simulink model "Tractor_Trailer_Flatness_Simulation"  (R2022b)
settings: Solver=ode4  StartTime=0.01  StopTime=20  FixedStep=0.01  RelTol=1e-3
InitFcn:
  | d0 = 1;
  | Dt=0.01;
  | 
  | %% if we want to "externalise" the trailer link from the car
  | a = 1.5;
  | 
  | %% distance between car and trailer
  | b = 2.5;
  | 
  | d1=b;
  | 
  | delay = 0.01;
  | 
  | %% delay with 0 signal before (to avoid instabilities before the "real" path following simulation")
  | del=2;
  | 
  | %% delay to sub above to chose starting using real value
  | dedel=1;
  | 
  | y0 = 0;
  | x0 = d1;
  | co=0;
  | 
  | the_pre=0;
  | the_pre_pre=0;
  | sdt=0.01;
  | 
  | ti_mod = 0.3;
  | 
  | phi0=pi;
  | 
  | %% Backward= pi, forward = 0
  | for_back=pi;
  | %%
  | 
  | %% Circle initial conditons forward
  | % for_back=0;
  | % dedel = 1.5;
  | % x_dot_init = 0;
  | % y_dot_init = 3;
  | % x_init = 0;
  | % y_init = 0;
  | % x0_init = b + del-dedel;
  | % y0_init = 0;
  | % theta0_init=for_back;
  | % theta1_init=0;
  | 
  | %% Circle initial conditons backward
  | % for_back=pi;
  | % dedel = 1.5;
  | % x_dot_init = 0;
  | % y_dot_init = 3;
  | % x_init = 0;
  | % y_init = 0;
  | % x0_init = -b;
  | % y0_init = 0;
  | % theta0_init=for_back;
  | % theta1_init=0;
  | 
  | %% func1 initial conditons
  | % x_dot_init = 1;
  | % y_dot_init = 0;
  | % x_init = 0;
  | % y_init = 0;
  | % x0_init = 0;
  | % y0_init = 0;
  | % theta0_init=0;
  | % theta1_init=0;
  | 
  | %% Wavy_up initial conditons
  | % x_dot_init = 0;
  | % y_dot_init = 0;
  | % x_init = 0;
  | % y_init = 0;
  | % x0_init = 0;
  | % y0_init = 0;
  | % theta0_init=0;
  | % theta1_init=0;
  | 
  | %% Backward Initial conditons for waving upward
  | % for_back=pi;
  | % x_dot_init = 1;
  | % y_dot_init = 0;
  | %
  | % x_init = 0;
  | % y_init = 0;
  | %
  | % %plant init
  | % x0_init = -b;
  | % y0_init = 0;
  | % theta0_init=for_back;
  | % theta1_init=0;
  | % del=pi;
  | 
  | %% Forward Initial conditons for waving upward
  | for_back=0;
  | x_dot_init = 1;
  | y_dot_init = 0;
  | 
  | x_init = 0;
  | y_init = 0;
  | 
  | %plant init
  | x0_init = b;
  | y0_init = 0;
  | theta0_init=for_back;
  | theta1_init=0;
  | del=pi;
  | 
  | 
  | %% Forward initial conditons for exp
  | % dedel=del;
  | % for_back=0;
  | % x_dot_init = 1;
  | % y_dot_init = 0;
  | % x_init = 0;
  | % y_init = 0;
  | % x0_init = 0;
  | % y0_init = 0;
  | % theta0_init=for_back;
  | % theta1_init=0;
  | 
  | %% Backward initial conditons for exp
  | % dedel=del-0.2;
  | % for_back=pi;
  | % x_dot_init = 1;
  | % y_dot_init = 0;
  | % x_init = 0;
  | % y_init = 0;
  | % x0_init = -b;
  | % y0_init = 0;
  | % theta0_init=for_back;
  | % theta1_init=0;
  | 
  | 
  | %% Cosinus initial conditons forward
  | % for_back=0;
  | % dedel=1;
  | % x_dot_init = 3;
  | % y_dot_init = 0;
  | % x_init = 0;
  | % y_init = 0;
  | % x0_init = b;
  | % y0_init = 0;
  | % theta0_init=for_back;
  | % theta1_init=0;
  | 
  | %% Cosinus initial conditons backward
  | % for_back=pi;
  | % dedel=1;
  | % x_dot_init = 3;
  | % y_dot_init = 0;
  | % x_init = 0;
  | % y_init = 0;
  | % x0_init = -b;
  | % y0_init = 0;
  | % theta0_init=for_back;
  | % theta1_init=0;
settings Model: Creator=chaudhuri  LastModifiedBy=Tugdual
settings ModelReferenceCC: EnableRefExpFcnMdlSchedulingChecks=on

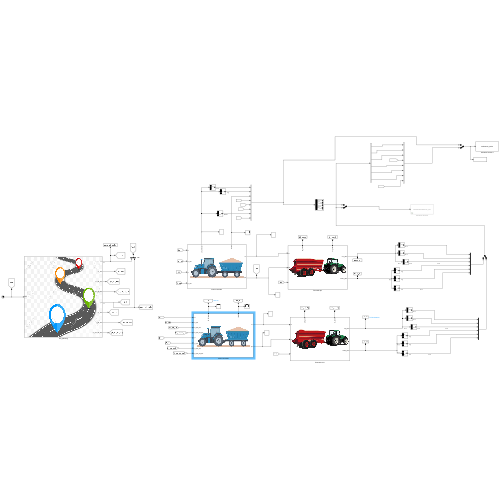
[thumbnail: Simulink's stored preview of the top-level diagram]
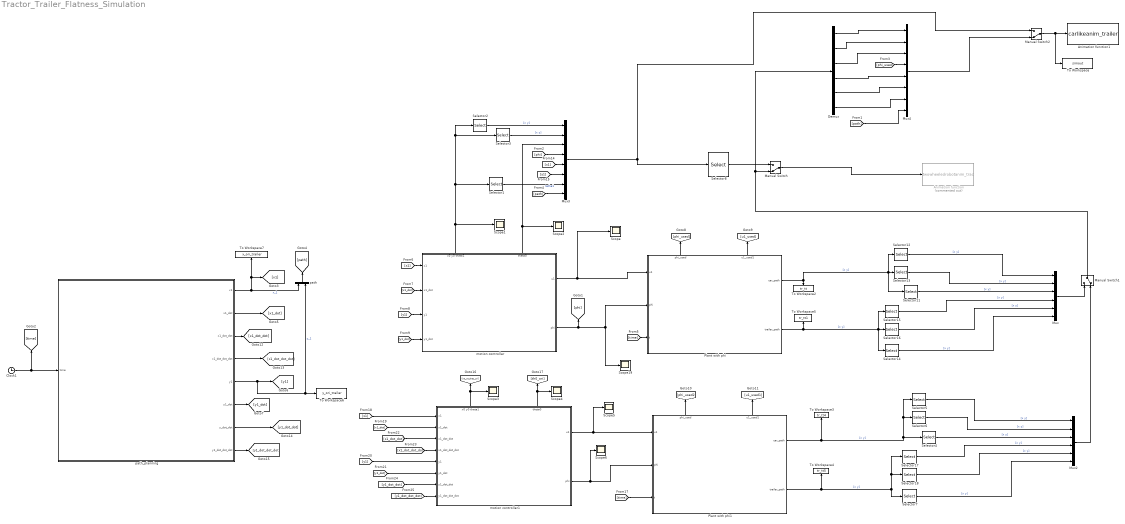
== system Tractor_Trailer_Flatness_Simulation ==
  Animation function : S-Function  Commented=on  FunctionName=twowheeledrobotanim_trac  SFunctionDeploymentMode=off  EnableBusSupport=off
  Animation function1 : S-Function  FunctionName=carlikeanim_trailer  SFunctionDeploymentMode=off  EnableBusSupport=off
  Clock1 : Clock
  Demux : Demux  Outputs=6
  Manual Switch : ManualSwitch  CurrentSetting=0
  Manual Switch1 : ManualSwitch  CurrentSetting=0
  Manual Switch2 : ManualSwitch  CurrentSetting=0
  Mux : Mux  Inputs=6
  Mux2 : Mux  Inputs=6
  Mux3 : Mux  Inputs=8
  Mux4 : Mux  Inputs=8
  Plant with phi : Subsystem
      settings: PortSchema="{\"entries\":[{\"content\":{\"sides\":[{\"content\":{\"connectorIds\":[\"In1\",\"In2\",\"In3\"]},\"type\":\"ConnectorPlacement.EquallySpacedRectSide\",\"uuid\":\"e7db4861-1c7b-44d0-8ae0-043891a2d65e\"},{\"content\":{\"connectorIds\":[\"Out1\",\"Out2\"],\"side\":\"RIGHT\"},\"type\":\"ConnectorPlacement.EquallySpacedRectSide\",\"uuid\":\"ca6953ca-f3e9-441a-9b66-bf77f2babfba\"},{\"content\":{\"connectorIds\":[\"Out3\",\"Out4\"],\"side\":\"TOP\"},\"type\":\"ConnectorPlacement.EquallySpacedRectSide\",\"uuid\":\"0653e744-f46f-49ca-b3b7-6a2721aef055\"}]},\"type\":\"ConnectorPlacement.EquallySpacedConnector\",\"uuid\":\"d05efadf-1bd4-4ab0-9eff-99e9b7844dfa\"}],\"packageUris\":[\"http://schema.mathworks.com/mf0/Connector/R2020b\"],\"version\":\"1.0\"}"
      mask Display: image('$imagefile'); % Use "Edit Image" on toolstrip to change.
  Plant with phi1 : Subsystem
      settings: PortSchema="{\"entries\":[{\"content\":{\"sides\":[{\"content\":{\"connectorIds\":[\"In1\",\"In2\",\"In3\"]},\"type\":\"ConnectorPlacement.EquallySpacedRectSide\",\"uuid\":\"e7db4861-1c7b-44d0-8ae0-043891a2d65e\"},{\"content\":{\"connectorIds\":[\"Out1\",\"Out2\"],\"side\":\"RIGHT\"},\"type\":\"ConnectorPlacement.EquallySpacedRectSide\",\"uuid\":\"ca6953ca-f3e9-441a-9b66-bf77f2babfba\"},{\"content\":{\"connectorIds\":[\"Out3\",\"Out4\"],\"side\":\"TOP\"},\"type\":\"ConnectorPlacement.EquallySpacedRectSide\",\"uuid\":\"0653e744-f46f-49ca-b3b7-6a2721aef055\"}]},\"type\":\"ConnectorPlacement.EquallySpacedConnector\",\"uuid\":\"d05efadf-1bd4-4ab0-9eff-99e9b7844dfa\"}],\"packageUris\":[\"http://schema.mathworks.com/mf0/Connector/R2020b\"],\"version\":\"1.0\"}"
      mask Display: image('$imagefile'); % Use "Edit Image" on toolstrip to change.
  Scope{,1..6,19} (8 alike) : Scope
  Selector{1,4,7,11,14} (5 alike) : Selector  InputPortWidth=3  IndexOptions=Index vector (dialog)  Indices=[3]  OutputSizes=1
  Selector{2,5,12,15,17} (5 alike) : Selector  InputPortWidth=3  IndexOptions=Index vector (dialog)  Indices=[1]  OutputSizes=1
  Selector{3,6,13,16,18} (5 alike) : Selector  InputPortWidth=3  IndexOptions=Index vector (dialog)  Indices=[2]  OutputSizes=1
  Selector8 : Selector  InputPortWidth=9  IndexOptions=Index vector (dialog)  Indices=[1 2 3 5 6 7]  OutputSizes=1
  To Workspace : ToWorkspace  VariableName=simout  SaveFormat=Timeseries  SampleTime=-1
  To Workspace2 : ToWorkspace  VariableName=tr_tt  SaveFormat=Timeseries  SampleTime=-1
  To Workspace3 : ToWorkspace  VariableName=tr_tt4  SaveFormat=Timeseries  SampleTime=-1
  To Workspace4 : ToWorkspace  VariableName=tr_tt5  SaveFormat=Timeseries  SampleTime=-1
  To Workspace5 : ToWorkspace  VariableName=tr_tt1  SaveFormat=Timeseries  SampleTime=-1
  To Workspace6 : ToWorkspace  VariableName=y_ori_trailer  SaveFormat=Timeseries  SampleTime=-1
      settings: Save2DSignal=2-D array (concatenate along first dimension)
  To Workspace7 : ToWorkspace  VariableName=x_ori_trailer  SaveFormat=Timeseries  SampleTime=-1
      settings: Save2DSignal=2-D array (concatenate along first dimension)
  motion controller : Subsystem
      settings: PortSchema="{\"entries\":[{\"content\":{\"sides\":[{\"content\":{\"connectorIds\":[\"In1\",\"In2\",\"In3\",\"In4\"]},\"type\":\"ConnectorPlacement.EquallySpacedRectSide\",\"uuid\":\"11bc3301-7ab6-4d38-8445-7de1e6050525\"},{\"content\":{\"connectorIds\":[\"Out1\",\"Out2\"],\"side\":\"RIGHT\"},\"type\":\"ConnectorPlacement.EquallySpacedRectSide\",\"uuid\":\"374bee85-8743-45f2-a60a-268bfdaad2ec\"},{\"content\":{\"connectorIds\":[\"Out3\",\"Out4\"],\"side\":\"TOP\"},\"type\":\"ConnectorPlacement.EquallySpacedRectSide\",\"uuid\":\"71c6a0a5-27e8-424b-8871-57b58ecd48a6\"}]},\"type\":\"ConnectorPlacement.EquallySpacedConnector\",\"uuid\":\"fb4e8639-9b4e-4508-bb82-15087a60f723\"}],\"packageUris\":[\"http://schema.mathworks.com/mf0/Connector/R2020b\"],\"version\":\"1.0\"}"
      mask Display: image('$imagefile'); % Use "Edit Image" on toolstrip to change.
  motion controller1 : Subsystem
      settings: PortSchema="{\"entries\":[{\"content\":{\"sides\":[{\"content\":{\"connectorIds\":[\"In1\",\"In2\",\"In3\",\"In4\",\"In5\",\"In6\",\"In7\",\"In8\"]},\"type\":\"ConnectorPlacement.EquallySpacedRectSide\",\"uuid\":\"11bc3301-7ab6-4d38-8445-7de1e6050525\"},{\"content\":{\"connectorIds\":[\"Out1\",\"Out2\"],\"side\":\"RIGHT\"},\"type\":\"ConnectorPlacement.EquallySpacedRectSide\",\"uuid\":\"374bee85-8743-45f2-a60a-268bfdaad2ec\"},{\"content\":{\"connectorIds\":[\"Out3\",\"Out4\"],\"side\":\"TOP\"},\"type\":\"ConnectorPlacement.EquallySpacedRectSide\",\"uuid\":\"71c6a0a5-27e8-424b-8871-57b58ecd48a6\"}]},\"type\":\"ConnectorPlacement.EquallySpacedConnector\",\"uuid\":\"fb4e8639-9b4e-4508-bb82-15087a60f723\"}],\"packageUris\":[\"http://schema.mathworks.com/mf0/Connector/R2020b\"],\"version\":\"1.0\"}"
      mask Display: image('$imagefile'); % Use "Edit Image" on toolstrip to change.
  path : Mux  Inputs=2
  path_planning : Subsystem
      mask Display: image('$imagefile'); % Use "Edit Image" on toolstrip to change.
  wires:
  Clock1/1 -> [time], path_planning/1(time)
  motion controller/2(phi) -> [phi], Plant with phi/2(phi), Scope19/1
  Plant with phi/1(car_path) -> Selector11/1, Selector12/1, Selector13/1, To Workspace2/1  "[x y]"
  Selector11/1 -> Mux/3  "[x y]"
  Selector12/1 -> Mux/1  "[x y]"
  Selector13/1 -> Mux/2  "[x y]"
  Selector16/1 -> Mux/5  "[x y]"
  Selector15/1 -> Mux/4  "[x y]"
  Plant with phi/2(trailer_path) -> Selector14/1, Selector15/1, Selector16/1, To Workspace5/1  "[x y]"
  Selector14/1 -> Mux/6  "[x y]"
  Manual Switch1/1 -> Demux/1, Manual Switch/2
  motion controller/1(u1) -> Plant with phi/1(u1), Scope/1
  motion controller/3(x0 y0 theta1) -> Scope1/1, Selector2/1, Selector3/1, Selector1/1
  Selector1/1 -> Mux3/7  "tetha1"
  Selector3/1 -> Mux3/2  "[x y]"
  Selector2/1 -> Mux3/1  "[x y]"
  Selector17/1 -> Mux2/4  "[x y]"
  Selector7/1 -> Mux2/6  "[x y]"
  Plant with phi1/2(trailer_path) -> To Workspace4/1, Selector18/1, Selector17/1, Selector7/1  "[x y]"
  Selector18/1 -> Mux2/5  "[x y]"
  Plant with phi1/1(car_path) -> Selector4/1, Selector5/1, Selector6/1, To Workspace3/1  "[x y]"
  Selector6/1 -> Mux2/2  "[x y]"
  Selector5/1 -> Mux2/1  "[x y]"
  Mux2/1 -> Manual Switch1/2
  Selector4/1 -> Mux2/3  "[x y]"
  Mux/1 -> Manual Switch1/1
  Manual Switch2/1 -> To Workspace/1, Animation function1/1
  Manual Switch/1 -> Animation function/1
  motion controller/4(theta0) -> Scope2/1, Mux3/3
  Mux4/1 -> Manual Switch2/2
  Mux3/1 -> Selector8/1, Manual Switch2/1
  Demux/1 -> Mux4/1
  Demux/2 -> Mux4/2
  Demux/3 -> Mux4/3
  Demux/4 -> Mux4/5
  Demux/5 -> Mux4/6
  Demux/6 -> Mux4/7
  path/1 -> [path]
  [path] -> Mux4/8
  [phi] -> Mux3/4
  [phi_used] -> Mux4/4
  [path] -> Mux3/8
  [time] -> Plant with phi/3(t)
  Selector8/1 -> Manual Switch/1
  [x1] -> Mux3/5
  [y1] -> Mux3/6
  [x1] -> motion controller/1(x1)
  [x1_dot] -> motion controller/2(x1_dot)
  [y1] -> motion controller/3(y1)
  [y1_dot] -> motion controller/4(y1_dot)
  path_planning/6(y1_dot) -> [y1_dot]
  path_planning/5(y1) -> To Workspace6/1, path/2, [y1]  "y_1"
  path_planning/2(x1_dot) -> [x1_dot]
  path_planning/1(x1) -> path/1, [x1], To Workspace7/1  "x_1"
  Plant with phi/3(phi_used) -> [phi_used]
  Plant with phi/4(u1_used1) -> [u1_used]
  motion controller1/1(u1) -> Scope5/1, Plant with phi1/1(u1)
  motion controller1/2(phi) -> Scope6/1, Plant with phi1/2(phi)
  [time] -> Plant with phi1/3(t)
  [x1_dot_dot] -> motion controller1/3(x1_dot_dot)
  [x1_dot] -> motion controller1/2(x1_dot)
  [x1] -> motion controller1/1(x1)
  [y1] -> motion controller1/5(y1)
  [y1_dot] -> motion controller1/6(y1_dot)
  [y1_dot_dot] -> motion controller1/7(y1_dot_dot)
  [y1_dot_dot_dot] -> motion controller1/8(y1_dot_dot_dot)
  [x1_dot_dot_dot] -> motion controller1/4(x1_dot_dot_dot)
  motion controller1/4(theta0) -> [th0_ori], Scope4/1
  motion controller1/3(x0 y0 theta1) -> Scope3/1, [x0_y0_the1_ori]
  Plant with phi1/4(u1_used1) -> [u1_used1]
  Plant with phi1/3(phi_used) -> [phi_used2]
  path_planning/8(y1_dot_dot_dot) -> [y1_dot_dot_dot]
  path_planning/7(y_dot_dot) -> [y1_dot_dot]
  path_planning/4(x1_dot_dot_dot) -> [x1_dot_dot_dot]
  path_planning/3(x1_dot_dot) -> [x1_dot_dot]

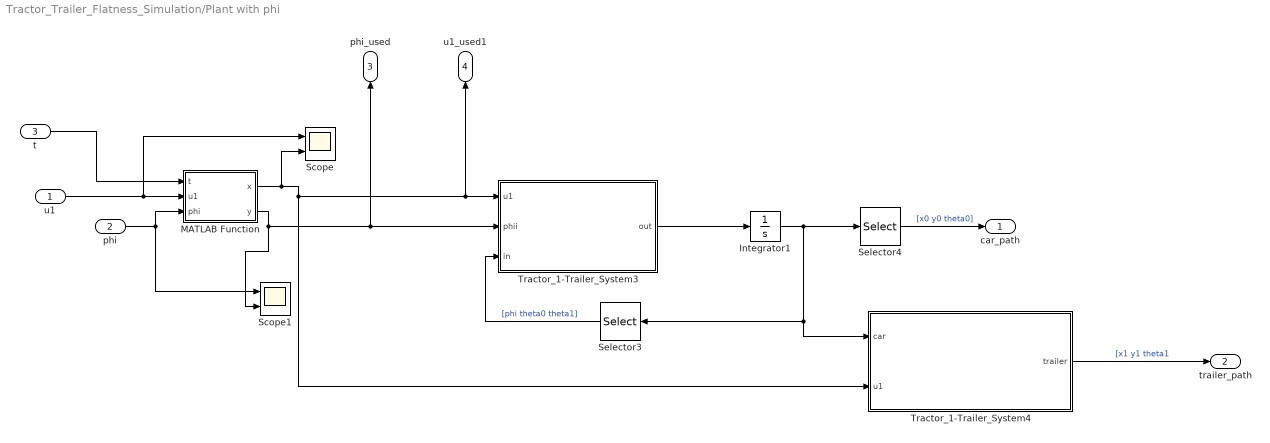
== system Tractor_Trailer_Flatness_Simulation/Plant with phi ==
  u1 : Inport
  phi : Inport  Port=2
  t : Inport  Port=3
  Integrator1 : Integrator  InitialCondition=[x0_init;y0_init;theta0_init;theta1_init]
  MATLAB Function : MATLAB Function  TreatAsAtomicUnit=on
  Scope : Scope  NumInputPorts=2
  Scope1 : Scope  NumInputPorts=2
  Selector3 : Selector  InputPortWidth=4  IndexOptions=Index vector (dialog)  Indices=[3 4]  OutputSizes=1
  Selector4 : Selector  InputPortWidth=4  IndexOptions=Index vector (dialog)  Indices=[1 2 3]  OutputSizes=1
  Tractor_1-Trailer_System3 : MATLAB Function  TreatAsAtomicUnit=on
  Tractor_1-Trailer_System4 : MATLAB Function  TreatAsAtomicUnit=on
  car_path : Outport
  trailer_path : Outport  Port=2
  phi_used : Outport  Port=3
  u1_used1 : Outport  Port=4
  wires:
  Tractor_1-Trailer_System4/1(trailer) -> trailer_path/1  "[x1 y1 theta1"
  Tractor_1-Trailer_System3/1(out) -> Integrator1/1
  Integrator1/1 -> Selector4/1, Tractor_1-Trailer_System4/1(car), Selector3/1
  Selector3/1 -> Tractor_1-Trailer_System3/3(in)  "[phi theta0 theta1]"
  Selector4/1 -> car_path/1  "[x0 y0 theta0]"
  MATLAB Function/2(y) -> Scope1/2, Tractor_1-Trailer_System3/2(phii), phi_used/1
  MATLAB Function/1(x) -> Scope/2, u1_used1/1, Tractor_1-Trailer_System3/1(u1), Tractor_1-Trailer_System4/2(u1)
  t/1 -> MATLAB Function/1(t)
  u1/1 -> Scope/1, MATLAB Function/2(u1)
  phi/1 -> Scope1/1, MATLAB Function/3(phi)

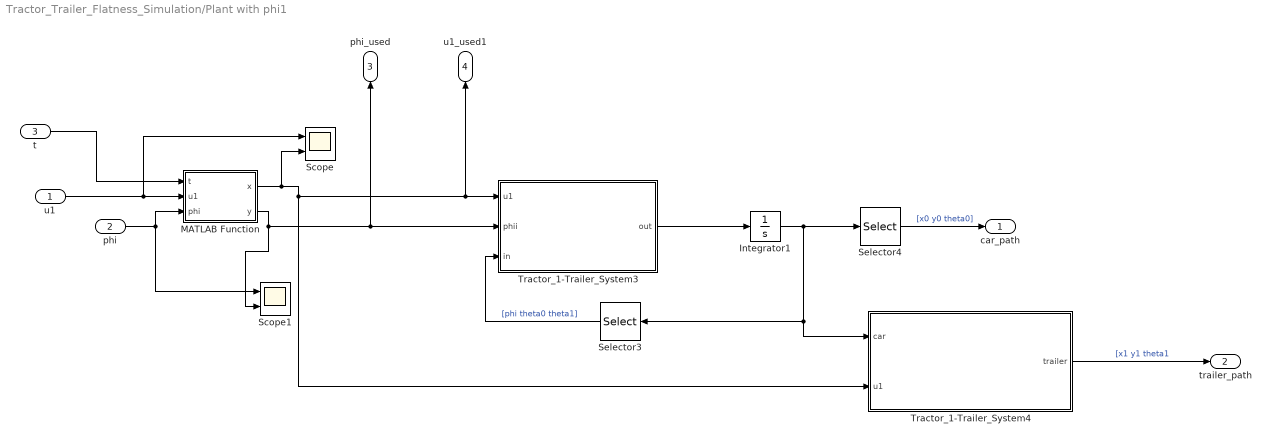
== system Tractor_Trailer_Flatness_Simulation/Plant with phi1 ==
  u1 : Inport
  phi : Inport  Port=2
  t : Inport  Port=3
  Integrator1 : Integrator  InitialCondition=[x0_init;y0_init;theta0_init;theta1_init]
  MATLAB Function : MATLAB Function  TreatAsAtomicUnit=on
  Scope : Scope  NumInputPorts=2
  Scope1 : Scope  NumInputPorts=2
  Selector3 : Selector  InputPortWidth=4  IndexOptions=Index vector (dialog)  Indices=[3 4]  OutputSizes=1
  Selector4 : Selector  InputPortWidth=4  IndexOptions=Index vector (dialog)  Indices=[1 2 3]  OutputSizes=1
  Tractor_1-Trailer_System3 : MATLAB Function  TreatAsAtomicUnit=on
  Tractor_1-Trailer_System4 : MATLAB Function  TreatAsAtomicUnit=on
  car_path : Outport
  trailer_path : Outport  Port=2
  phi_used : Outport  Port=3
  u1_used1 : Outport  Port=4
  wires:
  Tractor_1-Trailer_System4/1(trailer) -> trailer_path/1  "[x1 y1 theta1"
  Tractor_1-Trailer_System3/1(out) -> Integrator1/1
  Integrator1/1 -> Selector4/1, Tractor_1-Trailer_System4/1(car), Selector3/1
  Selector3/1 -> Tractor_1-Trailer_System3/3(in)  "[phi theta0 theta1]"
  Selector4/1 -> car_path/1  "[x0 y0 theta0]"
  MATLAB Function/2(y) -> Scope1/2, Tractor_1-Trailer_System3/2(phii), phi_used/1
  MATLAB Function/1(x) -> Scope/2, u1_used1/1, Tractor_1-Trailer_System3/1(u1), Tractor_1-Trailer_System4/2(u1)
  t/1 -> MATLAB Function/1(t)
  u1/1 -> Scope/1, MATLAB Function/2(u1)
  phi/1 -> Scope1/1, MATLAB Function/3(phi)

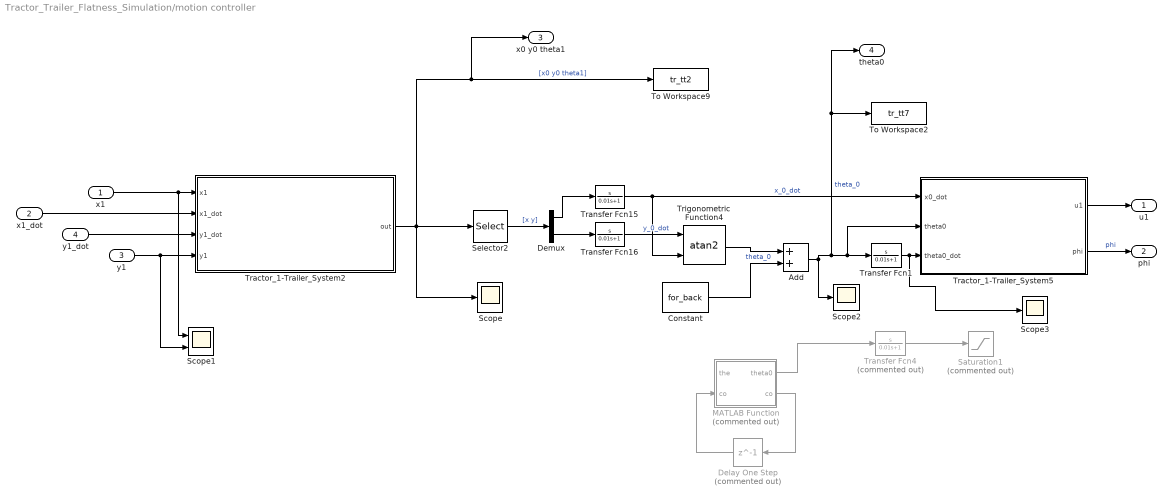
== system Tractor_Trailer_Flatness_Simulation/motion controller ==
  x1 : Inport
  x1_dot : Inport  Port=2
  y1 : Inport  Port=3
  y1_dot : Inport  Port=4
  Add : Sum
  Constant : Constant  Value=for_back
  Delay One Step : Delay  Commented=on  DelayLength=1
  Demux : Demux  Outputs=2
  MATLAB Function : MATLAB Function  Commented=on  TreatAsAtomicUnit=on
  Saturation1 : Saturate  Commented=on  UpperLimit=pi/4  LowerLimit=-pi/4
  Scope : Scope
  Scope1 : Scope  NumInputPorts=2
  Scope2 : Scope
  Scope3 : Scope
  Selector2 : Selector  InputPortWidth=3  IndexOptions=Index vector (dialog)  Indices=[1 2]  OutputSizes=1
  To Workspace2 : ToWorkspace  VariableName=tr_tt7  SaveFormat=Timeseries  SampleTime=-1
  To Workspace9 : ToWorkspace  VariableName=tr_tt2  SaveFormat=Timeseries  SampleTime=-1
  Tractor_1-Trailer_System2 : MATLAB Function  TreatAsAtomicUnit=on
  Tractor_1-Trailer_System5 : MATLAB Function  TreatAsAtomicUnit=on
  Transfer Fcn1 : TransferFcn  Numerator=[1 0]  Denominator=[0.01 1]
  Transfer Fcn15 : TransferFcn  Numerator=[1 0]  Denominator=[0.01 1]
  Transfer Fcn16 : TransferFcn  Numerator=[1 0]  Denominator=[0.01 1]
  Transfer Fcn4 : TransferFcn  Commented=on  Numerator=[1 0]  Denominator=[0.01 1]
  Trigonometric Function4 : Trigonometry  Operator=atan2
  u1 : Outport
  phi : Outport  Port=2
  x0 y0 theta1 : Outport  Port=3
  theta0 : Outport  Port=4
  wires:
  Selector2/1 -> Demux/1  "[x y]"
  Tractor_1-Trailer_System2/1(out) -> Scope/1, x0 y0 theta1/1, To Workspace9/1, Selector2/1  "[x0 y0 theta1]"
  Transfer Fcn16/1 -> Trigonometric Function4/1  "y_0_dot"
  Transfer Fcn1/1 -> Scope3/1, Tractor_1-Trailer_System5/3(theta0_dot)
  Add/1 -> theta0/1, To Workspace2/1, Tractor_1-Trailer_System5/2(theta0), Transfer Fcn1/1, Scope2/1  "theta_0"
  Transfer Fcn15/1 -> Tractor_1-Trailer_System5/1(x0_dot), Trigonometric Function4/2  "x_0_dot"
  Demux/2 -> Transfer Fcn16/1
  Demux/1 -> Transfer Fcn15/1
  Tractor_1-Trailer_System5/2(phi) -> phi/1  "phi"
  Tractor_1-Trailer_System5/1(u1) -> u1/1
  x1_dot/1 -> Tractor_1-Trailer_System2/2(x1_dot)
  Delay One Step/1 -> MATLAB Function/2("co ")
  MATLAB Function/1(theta0) -> Transfer Fcn4/1
  ? -> MATLAB Function/1(the)  "theta_0"
  MATLAB Function/2(co) -> Delay One Step/1
  Transfer Fcn4/1 -> Saturation1/1
  y1_dot/1 -> Tractor_1-Trailer_System2/3(y1_dot)
  y1/1 -> Scope1/2, Tractor_1-Trailer_System2/4(y1)
  x1/1 -> Scope1/1, Tractor_1-Trailer_System2/1(x1)
  Trigonometric Function4/1 -> Add/1  "theta_0"
  Constant/1 -> Add/2

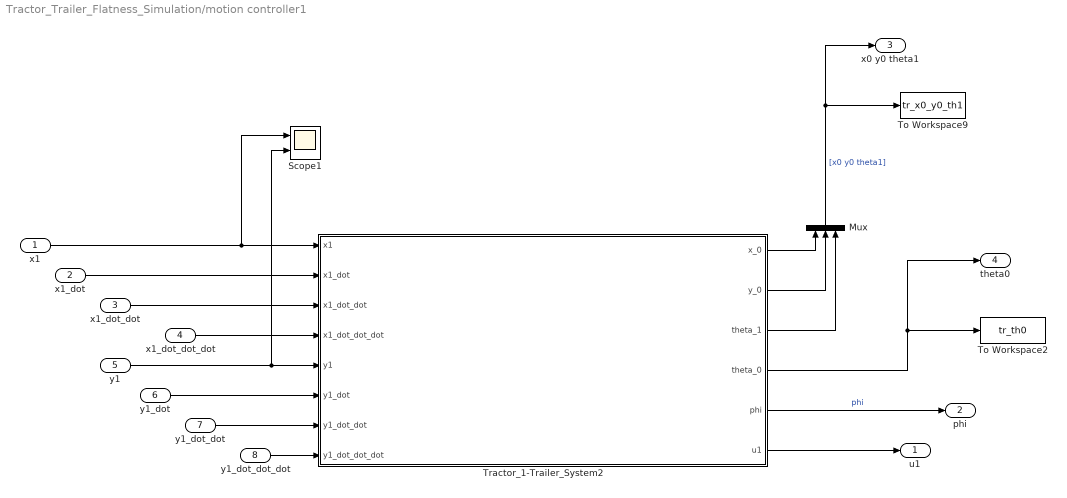
== system Tractor_Trailer_Flatness_Simulation/motion controller1 ==
  x1 : Inport
  x1_dot : Inport  Port=2
  x1_dot_dot : Inport  Port=3
  x1_dot_dot_dot : Inport  Port=4
  y1 : Inport  Port=5
  y1_dot : Inport  Port=6
  y1_dot_dot : Inport  Port=7
  y1_dot_dot_dot : Inport  Port=8
  Mux : Mux  Inputs=3
  Scope1 : Scope  NumInputPorts=2
  To Workspace2 : ToWorkspace  VariableName=tr_th0  SaveFormat=Timeseries  SampleTime=-1
  To Workspace9 : ToWorkspace  VariableName=tr_x0_y0_th1  SaveFormat=Timeseries  SampleTime=-1
  Tractor_1-Trailer_System2 : MATLAB Function  TreatAsAtomicUnit=on
  u1 : Outport
  phi : Outport  Port=2
  x0 y0 theta1 : Outport  Port=3
  theta0 : Outport  Port=4
  wires:
  Mux/1 -> x0 y0 theta1/1, To Workspace9/1  "[x0 y0 theta1]"
  Tractor_1-Trailer_System2/5(phi) -> phi/1  "phi"
  Tractor_1-Trailer_System2/6(u1) -> u1/1
  x1_dot/1 -> Tractor_1-Trailer_System2/2(x1_dot)
  y1_dot/1 -> Tractor_1-Trailer_System2/6(y1_dot)
  y1/1 -> Scope1/2, Tractor_1-Trailer_System2/5(y1)
  x1/1 -> Scope1/1, Tractor_1-Trailer_System2/1(x1)
  y1_dot_dot/1 -> Tractor_1-Trailer_System2/7(y1_dot_dot)
  y1_dot_dot_dot/1 -> Tractor_1-Trailer_System2/8(y1_dot_dot_dot)
  x1_dot_dot/1 -> Tractor_1-Trailer_System2/3(x1_dot_dot)
  x1_dot_dot_dot/1 -> Tractor_1-Trailer_System2/4(x1_dot_dot_dot)
  Tractor_1-Trailer_System2/3(theta_1) -> Mux/3
  Tractor_1-Trailer_System2/2(y_0) -> Mux/2
  Tractor_1-Trailer_System2/1(x_0) -> Mux/1
  Tractor_1-Trailer_System2/4(theta_0) -> To Workspace2/1, theta0/1

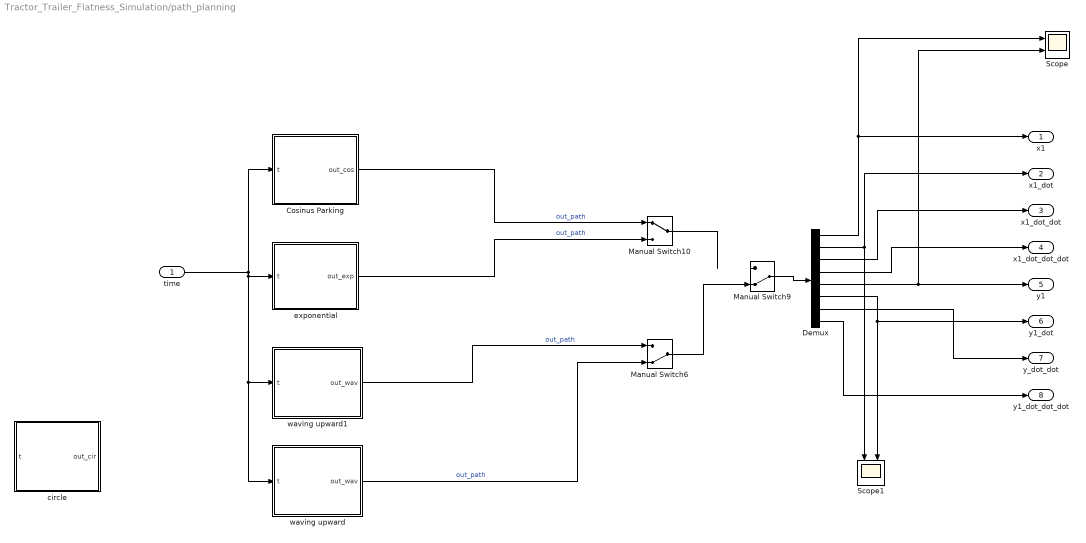
== system Tractor_Trailer_Flatness_Simulation/path_planning ==
  time : Inport
  Cosinus Parking : MATLAB Function  TreatAsAtomicUnit=on
  Demux : Demux  Outputs=8
  Manual Switch10 : ManualSwitch
  Manual Switch6 : ManualSwitch  CurrentSetting=0
  Manual Switch9 : ManualSwitch  CurrentSetting=0
  Scope : Scope  NumInputPorts=2
  Scope1 : Scope  NumInputPorts=2
  circle : MATLAB Function  TreatAsAtomicUnit=on
  exponential : MATLAB Function  TreatAsAtomicUnit=on
  waving upward : MATLAB Function  TreatAsAtomicUnit=on
  waving upward1 : MATLAB Function  TreatAsAtomicUnit=on
  x1 : Outport
  x1_dot : Outport  Port=2
  x1_dot_dot : Outport  Port=3
  x1_dot_dot_dot : Outport  Port=4
  y1 : Outport  Port=5
  y1_dot : Outport  Port=6
  y_dot_dot : Outport  Port=7
  y1_dot_dot_dot : Outport  Port=8
  wires:
  exponential/1(out_exp) -> Manual Switch10/2  "out_path"
  time/1 -> exponential/1(t), waving upward1/1(t), waving upward/1(t), Cosinus Parking/1(t)
  Demux/1 -> x1/1, Scope/1
  Demux/2 -> Scope1/1, x1_dot/1
  Demux/5 -> Scope/2, y1/1
  Demux/6 -> Scope1/2, y1_dot/1
  Manual Switch9/1 -> Demux/1
  waving upward/1(out_wav) -> Manual Switch6/2  "out_path"
  Cosinus Parking/1(out_cos) -> Manual Switch10/1  "out_path"
  Manual Switch10/1 -> ?
  waving upward1/1(out_wav) -> Manual Switch6/1  "out_path"
  Manual Switch6/1 -> Manual Switch9/2
  Demux/4 -> x1_dot_dot_dot/1
  Demux/3 -> x1_dot_dot/1
  Demux/7 -> y_dot_dot/1
  Demux/8 -> y1_dot_dot_dot/1

== matlab function Tractor_Trailer_Flatness_Simulation/Plant with phi/Tractor_1-Trailer_System4 ==
  data: trailer output; car input; d1 parameter; u1 input; for_back parameter
function trailer= fcn(car,d1,u1,for_back)

trailer = [car(1) - sign(u1)*d1*cos(car(4));car(2) - sign(u1)*d1*sin(car(4));car(4)+for_back];

== matlab function Tractor_Trailer_Flatness_Simulation/Plant with phi/MATLAB Function ==
  data: t input; x output; u1 input; y output; phi input; del parameter; dedel parameter; for_back parameter
function [x,y]= fcn(t,u1,phi,del, dedel, for_back)
if t<del-dedel
    if for_back == 0
        x=2;
    else
        x=-2;
    end
    y=for_back;
else
    x=u1;
    y=phi;
end

== matlab function Tractor_Trailer_Flatness_Simulation/Plant with phi1/Tractor_1-Trailer_System4 ==
  data: trailer output; car input; d1 parameter; u1 input; for_back parameter
function trailer= fcn(car,d1,u1,for_back)

trailer = [car(1) - sign(u1)*d1*cos(car(4));car(2) - sign(u1)*d1*sin(car(4));car(4)+for_back];

== matlab function Tractor_Trailer_Flatness_Simulation/path_planning/waving upward1 ==
  data: out_wav output; t input
function out_wav = fcn(t)
if t<0
    dddy=0;
    ddy=0;
    dy=0;
    y=0;
    x=2*t;
    dx=sqrt(4-dy^2);
    ddx=0;
    dddx=0;
else
dddy=-cos(t);
ddy=-sin(t);
dy=cos(t)-1;
y=sin(t) - t;
% x=sqrt(4*t-y^2);
x=sqrt(4*cos(t) - cos(2*t) + 5)*sec(t/2)*(2*asinh(sin(t/2)) + sin(t/2)* sqrt(6 - 2*cos(t)))/(2*sqrt(3 - cos(t)));

dx=sqrt(4-dy^2);
% ddx=sin(t);
ddx=(sin(t)*(cos(t) - 1))/sqrt(4 - (cos(t) - 1)^2);
% dddx=cos(t);

dddx=8*((sin(t/2))^2)*((cos(t/2))^4)*(cos(t) - 4)/((-((cos(t))^2) + 2*cos(t) + 3)^(3/2));
end
out_wav = [x,dx,ddx,dddx,y,dy,ddy,dddy];

== matlab function Tractor_Trailer_Flatness_Simulation/path_planning/circle ==
  data: out_cir output; t input
function out_cir= fcn(t)
if t<=1
    dx=3;
    x = 3*t;
    dy=0;
    y=0;
else
dy=-3*sin(t-1);
dx=3*cos(t-1);
x= 3 * sin(t-1) + 3;
y = 3*cos(t-1) - 3;
end
out_cir=[x,dx,y,dy];

== matlab function Tractor_Trailer_Flatness_Simulation/motion controller/Tractor_1-Trailer_System2 ==
  data: x1 input; x1_dot input; out output; y1_dot input; y1 input; d1 parameter; for_back parameter
function out = fcn(x1,x1_dot, y1_dot, y1, d1,for_back)
%% Trying to approximate tangente function with Leonhard Euler and then taylor series 
% the11=0;
% for n = 0:100
%     if n==0
%         the11=1*(y1_dot/x1_dot)/(1+(y1_dot/x1_dot));
%     else
%         prod=1;
%         for k = 1:n
%             prod=2*k*((y1_dot/x1_dot)^2)/((2*k+1)*(1+(y1_dot/x1_dot)^2));
%         end
%         the11=the11+prod*(y1_dot/x1_dot)/(1+(y1_dot/x1_dot)^2);
%     end
% end
% the111=0;
% for n = 0:100
%     the111=the111+((-1)^n)*((y1_dot/x1_dot)^(2*n+1))/(2*n+1);
% end
% the111=the111-for_back;
% the11=the11-for_back;

theta1 = atan2(y1_dot,x1_dot)-for_back;
% theta1 = atan2(y1,x1)-for_back;
y0 = y1 + d1*sin(theta1);
x0 = x1 + d1*cos(theta1);

out=[x0;y0;theta1];

== matlab function Tractor_Trailer_Flatness_Simulation/path_planning/Cosinus Parking ==
  data: t input; out_cos output
function out_cos = fcn(t)
if t<pi | t > 3*pi 
    x=2*t;
    y=0;
    dx=2;
    dy=0;
else
    x=2*t;
    y=cos(t)-cos(pi);
    dx=2;
    dy=-sin(t);
end
out_cos=[x, dx, y, dy];

%% tring to fix the jumps
% function out_cos = fcn(t)
% if t<pi | t > 3*pi 
%     x=2*t;
%     y=0;
%     dy=0;
%     dx=2;
% else
%     y=cos(t)-cos(pi);
%     x=sqrt(4*t^2-y^2);
%     dy=-sin(t);
%     dx=sqrt(4-dy^2);
% end
% out_cos=[x, dx, y, dy];

== matlab function Tractor_Trailer_Flatness_Simulation/motion controller/Tractor_1-Trailer_System5 ==
  data: u1 output; x0_dot input; theta0 input; phi output; theta0_dot input; d0 parameter
function [u1, phi]= fcn(x0_dot, theta0, theta0_dot, d0)
u1 = x0_dot/(cos(theta0));
phi = atan2(d0*theta0_dot,u1);

== matlab function Tractor_Trailer_Flatness_Simulation/motion controller/MATLAB Function ==
  data: the input; theta0 output; co input; co output
function [theta0,co]= fcn(the,co)
if u < -pi+0.005
    co = co + 2*pi;
end
theta0 = the - co;

== matlab function Tractor_Trailer_Flatness_Simulation/path_planning/waving upward ==
  data: out_wav output; t input
function out_wav = fcn(t)
if t<0
    dddy=0;
    ddy=0;
    dy=0;
    y=0;
    x=2*t;
    dx=sqrt(4-dy^2);
    ddx=0;
    dddx=0;
else
dddy=-cos(t);
ddy=-sin(t);
dy=cos(t)-1;
y=sin(t) - t;
% x=sqrt(4*t-y^2);
x=sqrt(4*cos(t) - cos(2*t) + 5)*sec(t/2)*(2*asinh(sin(t/2)) + sin(t/2)* sqrt(6 - 2*cos(t)))/(2*sqrt(3 - cos(t)));

dx=sqrt(4-dy^2);
% ddx=sin(t);
ddx=(sin(t)*(cos(t) - 1))/sqrt(4 - (cos(t) - 1)^2);
% dddx=cos(t);

dddx=8*((sin(t/2))^2)*((cos(t/2))^4)*(cos(t) - 4)/((-((cos(t))^2) + 2*cos(t) + 3)^(3/2));
end
out_wav = [x,dx,ddx,dddx,y,dy,ddy,dddy];

== matlab function Tractor_Trailer_Flatness_Simulation/path_planning/exponential ==
  data: t input; out_exp output; ti_mod parameter; dedel parameter; del parameter
% function out_exp = fcn(t,ti_mod)
% if t<3
%     y=exp(t*ti_mod)-1;
% %     y=exp(t-6);
%     x=2*t;
%     dx=2;
%     dy=ti_mod*exp(t*ti_mod);
% %     dy=exp(t-6);
% else
% %     y=exp(ti_mod*t+3*(1-ti_mod)-2);
%     y=exp(t*ti_mod)-1;
%     x=2*t;
%     dx=2;
%     dy=ti_mod*exp(t*ti_mod);
% %     dy=ti_mod*exp(ti_mod*t-6);
% end
% out_exp=[x,dx,y,dy];

function out_exp = fcn(t,ti_mod,dedel, del)
if t<del-dedel
    y=0;
%     y=exp(t-6);
    x=2*t;
    dx=2;
    dy=0;
%     dy=exp(t-6);
else
%     y=exp(ti_mod*t+3*(1-ti_mod)-2);
    y=exp((t-dedel)*ti_mod)-1;
    x=2*t;
    dx=2;
    dy=ti_mod*exp((t-dedel)*ti_mod);
%     dy=ti_mod*exp(ti_mod*t-6);
end
out_exp=[x,dx,y,dy];

== matlab function Tractor_Trailer_Flatness_Simulation/Plant with phi1/MATLAB Function ==
  data: t input; x output; u1 input; y output; phi input; del parameter; dedel parameter; for_back parameter
function [x,y]= fcn(t,u1,phi,del, dedel, for_back)
if t<del-dedel
    if for_back == 0
        x=2;
    else
        x=-2;
    end
    y=for_back;
else
    x=u1;
    y=phi;
end

== matlab function Tractor_Trailer_Flatness_Simulation/motion controller1/Tractor_1-Trailer_System2 ==
  data: x_0 output; y_0 output; x1 input; x1_dot input; x1_dot_dot input; x1_dot_dot_dot input; y1 input; theta_1 output; y1_dot input; y1_dot_dot input; y1_dot_dot_dot input; d1 parameter; for_back parameter; d0 parameter; theta_0 output; phi output; u1 output
function [x_0, y_0, theta_1, theta_0, phi,u1] = fcn(x1, x1_dot, x1_dot_dot, x1_dot_dot_dot, y1, y1_dot, y1_dot_dot, y1_dot_dot_dot, d1,for_back, d0)

theta_1 = atan2(y1_dot,x1_dot)-for_back;
 
 
y_0 = y1 + (d1*y1_dot)/((y1_dot^2/x1_dot^2 + 1)^(1/2)*x1_dot);
 
 
x_0 = x1 + d1/(y1_dot^2/x1_dot^2 + 1)^(1/2);
 
 
theta_0 = for_back + atan2((d1*x1_dot^2*y1_dot_dot + ((x1_dot^2 + y1_dot^2)/x1_dot^2)^(3/2)*x1_dot^3*y1_dot - d1*x1_dot*y1_dot*x1_dot_dot),(((x1_dot^2 + y1_dot^2)/x1_dot^2)^(3/2)*x1_dot^4 + d1*y1_dot^2*x1_dot_dot - d1*x1_dot*y1_dot*y1_dot_dot));
 
 
phi = atan2((d0*((((x1_dot^2 + y1_dot^2)/x1_dot^2)^(3/2)*x1_dot^3*y1_dot_dot - d1*y1_dot*x1_dot_dot^2 + d1*x1_dot^2*y1_dot_dot_dot + 3*((x1_dot^2 + y1_dot^2)/x1_dot^2)^(3/2)*x1_dot^2*y1_dot*x1_dot_dot + (3*((x1_dot^2 + y1_dot^2)/x1_dot^2)^(1/2)*((2*x1_dot*x1_dot_dot + 2*y1_dot*y1_dot_dot)/x1_dot^2 - (2*(x1_dot^2 + y1_dot^2)*x1_dot_dot)/x1_dot^3)*x1_dot^3*y1_dot)/2 - d1*x1_dot*y1_dot*x1_dot_dot_dot + d1*x1_dot*x1_dot_dot*y1_dot_dot)/(((x1_dot^2 + y1_dot^2)/x1_dot^2)^(3/2)*x1_dot^4 + d1*y1_dot^2*x1_dot_dot - d1*x1_dot*y1_dot*y1_dot_dot) - ((d1*x1_dot^2*y1_dot_dot + ((x1_dot^2 + y1_dot^2)/x1_dot^2)^(3/2)*x1_dot^3*y1_dot - d1*x1_dot*y1_dot*x1_dot_dot)*(4*((x1_dot^2 + y1_dot^2)/x1_dot^2)^(3/2)*x1_dot^3*x1_dot_dot - d1*x1_dot*y1_dot_dot^2 + (3*((x1_dot^2 + y1_dot^2)/x1_dot^2)^(1/2)*((2*x1_dot*x1_dot_dot + 2*y1_dot*y1_dot_dot)/x1_dot^2 - (2*(x1_dot^2 + y1_dot^2)*x1_dot_dot)/x1_dot^3)*x1_dot^4)/2 + d1*y1_dot^2*x1_dot_dot_dot - d1*x1_dot*y1_dot*y1_dot_dot_dot + d1*y1_dot*x1_dot_dot*y1_dot_dot))/(((x1_dot^2 + y1_dot^2)/x1_dot^2)^(3/2)*x1_dot^4 + d1*y1_dot^2*x1_dot_dot - d1*x1_dot*y1_dot*y1_dot_dot)^2)),((x1_dot - (d1*((2*y1_dot*y1_dot_dot)/x1_dot^2 - (2*y1_dot^2*x1_dot_dot)/x1_dot^3))/(2*(y1_dot^2/x1_dot^2 + 1)^(3/2)))*((d1*x1_dot^2*y1_dot_dot + ((x1_dot^2 + y1_dot^2)/x1_dot^2)^(3/2)*x1_dot^3*y1_dot - d1*x1_dot*y1_dot*x1_dot_dot)^2/(((x1_dot^2 + y1_dot^2)/x1_dot^2)^(3/2)*x1_dot^4 + d1*y1_dot^2*x1_dot_dot - d1*y1_dot_dot*y1_dot*x1_dot)^2 + 1)^(3/2)));
 
 
u1 = abs((x1_dot - (d1*((2*y1_dot*y1_dot_dot)/x1_dot^2 - (2*y1_dot^2*x1_dot_dot)/x1_dot^3))/(2*(y1_dot^2/x1_dot^2 + 1)^(3/2)))*((d1*x1_dot^2*y1_dot_dot + ((x1_dot^2 + y1_dot^2)/x1_dot^2)^(3/2)*x1_dot^3*y1_dot - d1*x1_dot*y1_dot*x1_dot_dot)^2/(((x1_dot^2 + y1_dot^2)/x1_dot^2)^(3/2)*x1_dot^4 + d1*y1_dot^2*x1_dot_dot - d1*x1_dot*y1_dot*y1_dot_dot)^2 + 1)^(1/2));
 

%% atan(y0/x0) : no derivative !
% 
% theta_1 = atan2(y1,x1);
%  
%  
% y_0 = y1 + (d1*y1)/(x1*(y1^2/x1^2 + 1)^(1/2));
%  
%  
% x_0 = x1 + d1/(y1^2/x1^2 + 1)^(1/2);
%  
%  
% theta_0 = atan2(y1,x1);
%  
%  
% phi = atan2((d0*x1*(x1*y1_dot - y1*x1_dot)),(x1^3*((x1^2 + y1^2)/x1^2)^(3/2)*x1_dot + d1*y1^2*x1_dot - d1*x1*y1*y1_dot));
%  
%  
% u1 = abs((x1^3*((x1^2 + y1^2)/x1^2)^(3/2)*x1_dot + d1*y1^2*x1_dot - d1*x1*y1*y1_dot)/(x1^3 + x1*y1^2));
%  

out = [theta_1, y_0, x_0, theta_0, phi,u1];

== matlab function Tractor_Trailer_Flatness_Simulation/Plant with phi1/Tractor_1-Trailer_System3 ==
  data: out output; u1 input; phii input; in input; a parameter; b parameter; d0 parameter; d1 parameter
function out = fcn(u1, phii, in, a, b, d0, d1)

phi = phii;
theta0 = in(1);
theta1 = in(2);

x0_dot = cos(theta0)*u1;
y0_dot = sin(theta0)*u1;

theta0_dot = (1/d0)*tan(phi)*u1;
%theta1_dot = (1/b)*((a/d0)*tan(phi)*cos(theta0 - theta1) - sin(theta0 - theta1))*u1;
% theta1_dot = (1/d1)*cos(theta0 - theta1)*sin(theta0-theta1)*u1;
% theta1_dot = (1/d1)*((a/d0)*tan(phi)*cos(theta0 - theta1) - sin(theta0 - theta1))*u1;
theta1_dot = (1/d1)*(sin(theta0 - theta1))*u1*sign(u1);

out = [x0_dot;y0_dot;theta0_dot;theta1_dot];

== matlab function Tractor_Trailer_Flatness_Simulation/Plant with phi/Tractor_1-Trailer_System3 ==
  data: out output; u1 input; phii input; in input; a parameter; b parameter; d0 parameter; d1 parameter
function out = fcn(u1, phii, in, a, b, d0, d1)

phi = phii;
theta0 = in(1);
theta1 = in(2);

x0_dot = cos(theta0)*u1;
y0_dot = sin(theta0)*u1;

theta0_dot = (1/d0)*tan(phi)*u1;
%theta1_dot = (1/b)*((a/d0)*tan(phi)*cos(theta0 - theta1) - sin(theta0 - theta1))*u1;
% theta1_dot = (1/d1)*cos(theta0 - theta1)*sin(theta0-theta1)*u1;
% theta1_dot = (1/d1)*((a/d0)*tan(phi)*cos(theta0 - theta1) - sin(theta0 - theta1))*u1;
theta1_dot = (1/d1)*(sin(theta0 - theta1))*u1*sign(u1);

out = [x0_dot;y0_dot;theta0_dot;theta1_dot];
